simulink model "DC_velo_con"  (R2024a)
settings: Solver=ode45  StartTime=0.0  StopTime=0.4  RelTol=1e-4
values from neighbouring files (symbols this model uses):
  K = Te_rated/Ia_rated    (= 0.424752712124)    [set_DC_motor_param.m]
  Kas = 1/Kps    (= 8.42763317706)    [set_DC_motor_param.m]
  Kis = J*Wcs*Wcs/(5*Te_rated)    (= 11.8657276485)    [set_DC_motor_param.m]
  Kps = J*Wcs/Te_rated    (= 0.118657276485)    [set_DC_motor_param.m]
  Te_rated = Power/Wm_rated    (= 10.6188178031)    [set_DC_motor_param.m]
settings Model: Creator=CDSL-2  LastModifiedBy=CDSL-2

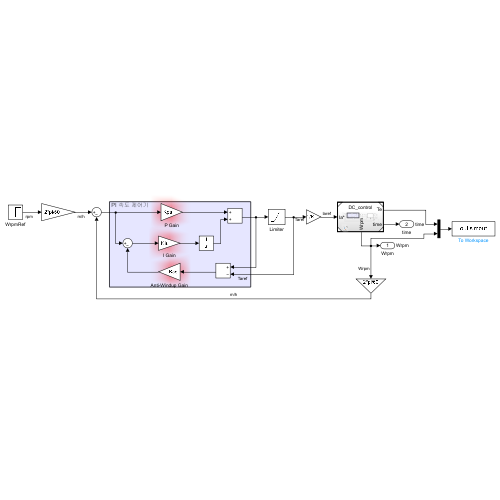
[thumbnail: Simulink's stored preview of the top-level diagram]
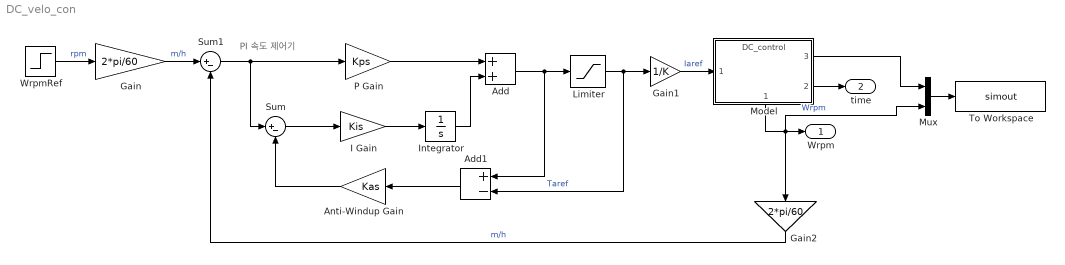
== system DC_velo_con ==
  note: PI 속도 제어기
  Add : Sum
  Add1 : Sum  Inputs=+-
  Anti-Windup Gain : Gain  Gain=Kas
  Gain : Gain  Gain=2*pi/60
  Gain1 : Gain  Gain=1/K
  Gain2 : Gain  Gain=2*pi/60
  I Gain : Gain  Gain=Kis
  Integrator : Integrator
  Limiter : Saturate  UpperLimit=Te_rated  LowerLimit=-Te_rated
  Model : ModelReference  ModelNameDialog=DC_control.slx  SimulationMode=Normal  ModelReferenceVersion=1.17
      settings: PortSchema="{\"entries\":[{\"content\":{\"sides\":[{\"content\":{\"connectorIds\":[\"In1\"]},\"type\":\"ConnectorPlacement.EquallySpacedRectSide\",\"uuid\":\"7ebac5d3-aa0f-4dc9-b259-8fac6335bc7b\"},{\"content\":{\"connectorIds\":[\"Out3\",\"Out2\"],\"side\":\"RIGHT\"},\"type\":\"ConnectorPlacement.EquallySpacedRectSide\",\"uuid\":\"9b2a9b96-6af6-4731-bab2-ea0927b548b6\"},{\"content\":{\"side\":\"TOP\"},\"type\":\"ConnectorPlacement.EquallySpacedRectSide\",\"uuid\":\"8b5fe18f-f2af-4690-ad81-2f0c010ef420\"},{\"content\":{\"connectorIds\":[\"Out1\"],\"side\":\"BOTTOM\"},\"type\":\"ConnectorPlacement.EquallySpacedRectSide\",\"uuid\":\"e686170b-4d67-4d8f-92c3-4ef4787df2cb\"}]},\"type\":\"ConnectorPlacement.EquallySpacedConnector\",\"uuid\":\"dc390c58-2f0f-4178-b726-6c1821c52cc3\"}],\"packageUris\":[\"http://schema.mathworks.com/mf0/Connector/R2020b\"],\"version\":\"1.0\"}"
  Mux : Mux  Inputs=2
  P Gain : Gain  Gain=Kps
  Sum : Sum  Inputs=|+-
  Sum1 : Sum  Inputs=|+-
  To Workspace : ToWorkspace  VariableName=simout  SaveFormat=Timeseries  SampleTime=-1
  WrpmRef : Step  Time=0.05  After=2500  SampleTime=0
  Wrpm : Outport  SignalName=Wrpm  Unit=rpm
  time : Outport  Port=2  SignalName=time  Unit=sec
  wires:
  I Gain/1 -> Integrator/1
  Integrator/1 -> Add/2
  P Gain/1 -> Add/1
  Sum/1 -> I Gain/1
  Sum1/1 -> Sum/1, P Gain/1
  Add1/1 -> Anti-Windup Gain/1
  Add/1 -> Add1/1, Limiter/1
  Anti-Windup Gain/1 -> Sum/2
  WrpmRef/1 -> Gain/1  "rpm"
  Gain/1 -> Sum1/1  "m/h"
  Gain1/1 -> Model/1  "Iaref"
  Limiter/1 -> Add1/2, Gain1/1  "Taref"
  Model/1 -> Mux/2, Gain2/1, Wrpm/1  "Wrpm"
  Gain2/1 -> Sum1/2  "m/h"
  Model/2 -> time/1
  Mux/1 -> To Workspace/1
  Model/3 -> Mux/1
